simulink model "prelab2simulink"  (R2014a)
settings: Solver=ode45  StartTime=0.0  StopTime=3.0  MaxStep=.001  RelTol=1e-3
settings Model: Creator=Matthew  LastModifiedBy=Matthew
settings DataIOCC: LimitDataPoints=off

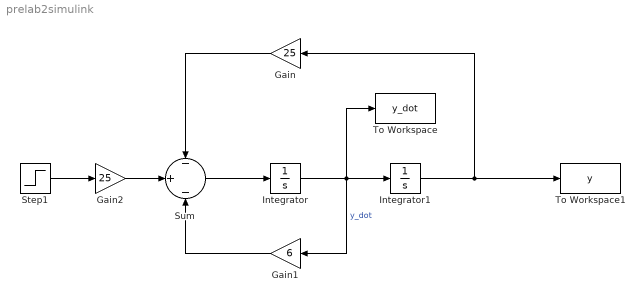
== system prelab2simulink ==
  Gain : Gain  Gain=25
  Gain1 : Gain  Gain=6
  Gain2 : Gain  Gain=25
  Integrator : Integrator
  Integrator1 : Integrator
  Step1 : Step  Time=0  SampleTime=0
  Sum : Sum  Inputs=-|+|-
  To Workspace : ToWorkspace  VariableName=y_dot  SampleTime=-1
  To Workspace1 : ToWorkspace  VariableName=y  SampleTime=-1
  wires:
  Gain1/1 -> Sum/3
  Gain/1 -> Sum/1
  Integrator/1 -> To Workspace/1, Gain1/1, Integrator1/1  "y_dot"
  Sum/1 -> Integrator/1
  Integrator1/1 -> To Workspace1/1, Gain/1
  Step1/1 -> Gain2/1
  Gain2/1 -> Sum/2
